simulink subsystem "ApplicationMotorSwapSysControl"  (R2024b)
settings: Solver=VariableStepAuto  StartTime=0.0  StopTime=10.0  RelTol=1e-3
values from neighbouring files (symbols this model uses):
  Ts = T_pwm    [mcbMotorSwapData.m]
  Ts_speed = 10*Ts    [mcbMotorSwapData.m]
undefined symbols (not defined in the file or in its folder): Per, Unit
libraries: simulink x2, mcbcomputeparameterlib x2, mcbcontrollergainlib x1
settings Model: Creator=The MathWorks, Inc.  LastModifiedBy=snarayan
settings RTWCC: GPUComputeCapability=3.5

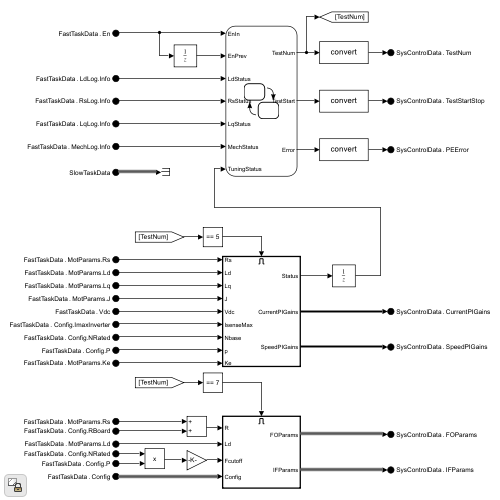
[thumbnail: Simulink's stored preview of the top-level diagram]
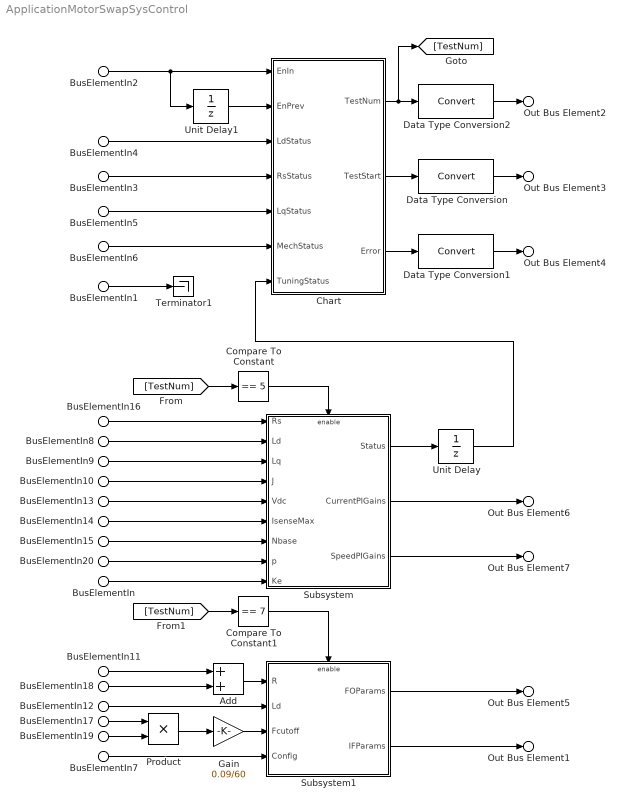
== system ApplicationMotorSwapSysControl ==
  BusElementIn2 : Inport  PortName=FastTaskData  Element=En
  BusElementIn3 : Inport  PortName=FastTaskData  Element=RsLog.Info
  BusElementIn4 : Inport  PortName=FastTaskData  Element=LdLog.Info
  BusElementIn5 : Inport  PortName=FastTaskData  Element=LqLog.Info
  BusElementIn6 : Inport  PortName=FastTaskData  Element=MechLog.Info
  BusElementIn11 : Inport  PortName=FastTaskData  Element=MotParams.Rs
  BusElementIn16 : Inport  PortName=FastTaskData  Element=MotParams.Rs
  BusElementIn8 : Inport  PortName=FastTaskData  Element=MotParams.Ld
  BusElementIn12 : Inport  PortName=FastTaskData  Element=MotParams.Ld
  BusElementIn9 : Inport  PortName=FastTaskData  Element=MotParams.Lq
  BusElementIn10 : Inport  PortName=FastTaskData  Element=MotParams.J
  BusElementIn : Inport  PortName=FastTaskData  Element=MotParams.Ke
  BusElementIn13 : Inport  PortName=FastTaskData  Element=Vdc
  BusElementIn7 : Inport  PortName=FastTaskData  Element=Config
  BusElementIn14 : Inport  PortName=FastTaskData  Element=Config.ImaxInverter
  BusElementIn15 : Inport  PortName=FastTaskData  Element=Config.NRated
  BusElementIn17 : Inport  PortName=FastTaskData  Element=Config.NRated
  BusElementIn18 : Inport  PortName=FastTaskData  Element=Config.RBoard
  BusElementIn19 : Inport  PortName=FastTaskData  Element=Config.P
  BusElementIn20 : Inport  PortName=FastTaskData  Element=Config.P
  BusElementIn1 : Inport  Port=2  PortName=SlowTaskData
  Add : Sum  RndMeth=Simplest  OutDataTypeStr=Inherit: Same as first input
  Chart : Stateflow chart  TreatAsAtomicUnit=on
  Compare To Constant : simulink/Logic and Bit Operations/Compare To Constant  relop===  const=5  OutDataTypeStr=boolean
  Compare To Constant1 : simulink/Logic and Bit Operations/Compare To Constant  relop===  const=7  OutDataTypeStr=boolean
  Data Type Conversion : DataTypeConversion  RndMeth=Simplest  SaturateOnIntegerOverflow=off
  Data Type Conversion1 : DataTypeConversion  RndMeth=Simplest  SaturateOnIntegerOverflow=off
  Data Type Conversion2 : DataTypeConversion  RndMeth=Simplest  SaturateOnIntegerOverflow=off
  Gain : Gain  Gain=0.09/60  RndMeth=Simplest  OutDataTypeStr=Inherit: Same as input
  Product : Product
  Subsystem : Subsystem
  Subsystem1 : Subsystem
  Terminator1 : Terminator
  Unit Delay : UnitDelay  SampleTime=-1  HasFrameUpgradeWarning=on
  Unit Delay1 : UnitDelay  SampleTime=-1  HasFrameUpgradeWarning=on
  Out Bus Element2 : Outport  PortName=SysControlData  Element=TestNum
  Out Bus Element3 : Outport  PortName=SysControlData  Element=TestStartStop
  Out Bus Element4 : Outport  PortName=SysControlData  Element=PEError
  Out Bus Element5 : Outport  PortName=SysControlData  Element=FOParams
  Out Bus Element6 : Outport  PortName=SysControlData  Element=CurrentPIGains
  Out Bus Element7 : Outport  PortName=SysControlData  Element=SpeedPIGains
  Out Bus Element1 : Outport  PortName=SysControlData  Element=IFParams
  wires:
  BusElementIn1/1 -> Terminator1/1
  BusElementIn2/1 -> Chart/1(EnIn), Unit Delay1/1
  Unit Delay1/1 -> Chart/2(EnPrev)
  Chart/1(TestNum) -> Data Type Conversion2/1, [TestNum]
  Chart/2(TestStart) -> Data Type Conversion/1
  BusElementIn3/1 -> Chart/4(RsStatus)
  BusElementIn4/1 -> Chart/3(LdStatus)
  BusElementIn5/1 -> Chart/5(LqStatus)
  BusElementIn6/1 -> Chart/6(MechStatus)
  Chart/3(Error) -> Data Type Conversion1/1
  BusElementIn8/1 -> Subsystem/2(Ld)
  BusElementIn9/1 -> Subsystem/3(Lq)
  BusElementIn10/1 -> Subsystem/4(J)
  Subsystem/1(Status) -> Unit Delay/1
  Unit Delay/1 -> Chart/7(TuningStatus)
  Data Type Conversion/1 -> Out Bus Element3/1
  Data Type Conversion1/1 -> Out Bus Element4/1
  Data Type Conversion2/1 -> Out Bus Element2/1
  BusElementIn11/1 -> Add/1
  BusElementIn12/1 -> Subsystem1/2(Ld)
  Subsystem1/1(FOParams) -> Out Bus Element5/1
  [TestNum] -> Compare To Constant/1
  Compare To Constant/1 -> Subsystem/Enable
  [TestNum] -> Compare To Constant1/1
  Compare To Constant1/1 -> Subsystem1/Enable
  Add/1 -> Subsystem1/1(R)
  BusElementIn13/1 -> Subsystem/5(Vdc)
  Product/1 -> Gain/1
  Gain/1 -> Subsystem1/3(Fcutoff)
  Subsystem/2(CurrentPIGains) -> Out Bus Element6/1
  Subsystem/3(SpeedPIGains) -> Out Bus Element7/1
  Subsystem1/2(IFParams) -> Out Bus Element1/1
  BusElementIn7/1 -> Subsystem1/4(Config)
  BusElementIn14/1 -> Subsystem/6(IsenseMax)
  BusElementIn15/1 -> Subsystem/7(Nbase)
  BusElementIn16/1 -> Subsystem/1(Rs)
  BusElementIn18/1 -> Add/2
  BusElementIn19/1 -> Product/2
  BusElementIn17/1 -> Product/1
  BusElementIn/1 -> Subsystem/9(Ke)
  BusElementIn20/1 -> Subsystem/8(p)

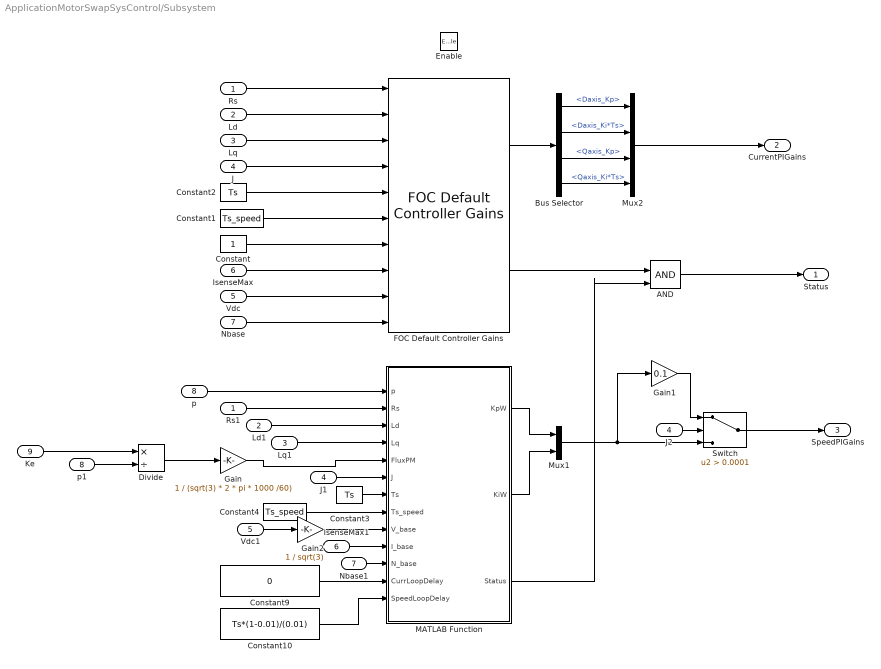
== system ApplicationMotorSwapSysControl/Subsystem ==
  Rs : Inport
  Ld : Inport  Port=2
  Lq : Inport  Port=3
  J : Inport  Port=4
  Vdc : Inport  Port=5
  IsenseMax : Inport  Port=6
  Nbase : Inport  Port=7
  p : Inport  Port=8
  Ke : Inport  Port=9
  Enable : EnablePort
  AND : Logic  IconShape=distinctive  AllPortsSameDT=off  OutDataTypeStr=boolean
  Bus Selector : BusSelector  OutputSignals=Daxis_Kp,Daxis_Ki*Ts,Qaxis_Kp,Qaxis_Ki*Ts
  Constant : Constant  OutDataTypeStr=dataType
  Constant1 : Constant  Value=Ts_speed  OutDataTypeStr=dataType
  Constant10 : Constant  Value=Ts*(1-0.01)/(0.01)  OutDataTypeStr=dataType
  Constant2 : Constant  Value=Ts  OutDataTypeStr=dataType
  Constant3 : Constant  Value=Ts  OutDataTypeStr=dataType
  Constant4 : Constant  Value=Ts_speed  OutDataTypeStr=dataType
  Constant9 : Constant  Value=0  OutDataTypeStr=dataType
  Divide : Product  Inputs=*/  RndMeth=Simplest  OutDataTypeStr=Inherit: Same as first input
  FOC Default Controller Gains : mcbcontrollergainlib/FOC Default Controller Gains  motorSelection=PMSM  unitType=Per-Unit  outCurrentControlGain=on  outFWCGain=off  outSpeedControlGain=on  externalDelay=off  currentSensorDelay=50e-6  speedSensorDelay=50e-6  speedFilterDelay=0.02
  Gain : Gain  Gain=1 / (sqrt(3) * 2 * pi * 1000 /60)  RndMeth=Simplest  OutDataTypeStr=Inherit: Same as input
  Gain1 : Gain  Gain=0.1  RndMeth=Simplest  OutDataTypeStr=Inherit: Same as input
  Gain2 : Gain  Gain=1 / sqrt(3)  RndMeth=Simplest  OutDataTypeStr=Inherit: Same as input
  IsenseMax1 : InportShadow  Port=6
  J1 : InportShadow  Port=4
  J2 : InportShadow  Port=4
  Ld1 : InportShadow  Port=2
  Lq1 : InportShadow  Port=3
  MATLAB Function : MATLAB Function  TreatAsAtomicUnit=on
  Mux1 : Mux  Inputs=2
  Mux2 : Mux
  Nbase1 : InportShadow  Port=7
  Rs1 : InportShadow
  Switch : Switch  Criteria=u2 > Threshold  Threshold=0.0001  SaturateOnIntegerOverflow=off  InputSameDT=off
  Vdc1 : InportShadow  Port=5
  p1 : InportShadow  Port=8
  Status : Outport
  CurrentPIGains : Outport  Port=2
  SpeedPIGains : Outport  Port=3
  wires:
  Gain1/1 -> Switch/1
  J2/1 -> Switch/2
  Switch/1 -> SpeedPIGains/1
  Bus Selector/4 -> Mux2/4  "<Qaxis_Ki*Ts>"
  Bus Selector/3 -> Mux2/3  "<Qaxis_Kp>"
  Bus Selector/2 -> Mux2/2  "<Daxis_Ki*Ts>"
  Bus Selector/1 -> Mux2/1  "<Daxis_Kp>"
  FOC Default Controller Gains/2 -> AND/1
  MATLAB Function/2(KiW) -> Mux1/2
  MATLAB Function/1(KpW) -> Mux1/1
  FOC Default Controller Gains/1 -> Bus Selector/1
  Gain2/1 -> MATLAB Function/9(V_base)
  AND/1 -> Status/1
  Vdc1/1 -> Gain2/1
  p1/1 -> Divide/2
  Ke/1 -> Divide/1
  p/1 -> MATLAB Function/1(p)
  Gain/1 -> MATLAB Function/5(FluxPM)
  Divide/1 -> Gain/1
  Nbase1/1 -> MATLAB Function/11(N_base)
  IsenseMax1/1 -> MATLAB Function/10(I_base)
  Constant4/1 -> MATLAB Function/8(Ts_speed)
  Constant3/1 -> MATLAB Function/7(Ts)
  J1/1 -> MATLAB Function/6(J)
  Lq1/1 -> MATLAB Function/4(Lq)
  Ld1/1 -> MATLAB Function/3(Ld)
  Rs1/1 -> MATLAB Function/2(Rs)
  Constant9/1 -> MATLAB Function/12(CurrLoopDelay)
  Constant10/1 -> MATLAB Function/13(SpeedLoopDelay)
  MATLAB Function/3(Status) -> AND/2
  Mux1/1 -> Gain1/1, Switch/3
  Mux2/1 -> CurrentPIGains/1
  Lq/1 -> FOC Default Controller Gains/3
  Nbase/1 -> FOC Default Controller Gains/10
  Vdc/1 -> FOC Default Controller Gains/9
  J/1 -> FOC Default Controller Gains/4
  Ld/1 -> FOC Default Controller Gains/2
  Constant2/1 -> FOC Default Controller Gains/5
  Constant/1 -> FOC Default Controller Gains/7
  IsenseMax/1 -> FOC Default Controller Gains/8
  Constant1/1 -> FOC Default Controller Gains/6
  Rs/1 -> FOC Default Controller Gains/1

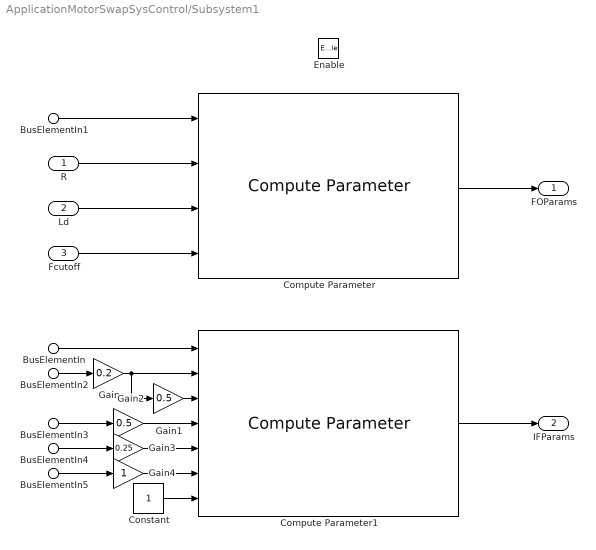
== system ApplicationMotorSwapSysControl/Subsystem1 ==
  R : Inport
  Ld : Inport  Port=2
  Fcutoff : Inport  Port=3
  BusElementIn : Inport  Port=4  PortName=Config  Element=P
  BusElementIn1 : Inport  Port=4  PortName=Config  Element=P
  BusElementIn2 : Inport  Port=4  PortName=Config  Element=NRated
  BusElementIn4 : Inport  Port=4  PortName=Config  Element=NRated
  BusElementIn3 : Inport  Port=4  PortName=Config  Element=IRated
  BusElementIn5 : Inport  Port=4  PortName=Config  Element=IRated
  Enable : EnablePort
  Compute Parameter : mcbcomputeparameterlib/Compute Parameter  PathOfCompatibleBlock=Microcontroller/ApplicationFastTask/FluxObserver/Flux Observer
  Compute Parameter1 : mcbcomputeparameterlib/Compute Parameter  PathOfCompatibleBlock=Microcontroller/ApplicationFastTask/FOCRun/IFController/I-F Controller
  Constant : Constant  OutDataTypeStr=dataType
  Gain : Gain  Gain=0.2  RndMeth=Simplest  OutDataTypeStr=Inherit: Same as input
  Gain1 : Gain  Gain=0.5  RndMeth=Simplest  OutDataTypeStr=Inherit: Same as input
  Gain2 : Gain  Gain=0.5  RndMeth=Simplest  OutDataTypeStr=Inherit: Same as input
  Gain3 : Gain  Gain=0.25  RndMeth=Simplest  OutDataTypeStr=Inherit: Same as input
  Gain4 : Gain  RndMeth=Simplest  OutDataTypeStr=Inherit: Same as input
  FOParams : Outport
  IFParams : Outport  Port=2
  wires:
  Gain4/1 -> Compute Parameter1/6
  BusElementIn5/1 -> Gain4/1
  Constant/1 -> Compute Parameter1/7
  BusElementIn4/1 -> Gain3/1
  Gain3/1 -> Compute Parameter1/5
  Gain2/1 -> Compute Parameter1/4
  BusElementIn3/1 -> Gain2/1
  Gain1/1 -> Compute Parameter1/3
  Gain/1 -> Gain1/1, Compute Parameter1/2
  BusElementIn2/1 -> Gain/1
  Compute Parameter1/1 -> IFParams/1
  BusElementIn/1 -> Compute Parameter1/1
  BusElementIn1/1 -> Compute Parameter/1
  Ld/1 -> Compute Parameter/3
  Compute Parameter/1 -> FOParams/1
  Fcutoff/1 -> Compute Parameter/4
  R/1 -> Compute Parameter/2

== matlab function ApplicationMotorSwapSysControl/Subsystem/MATLAB Function ==
  data: p input; KpW output; KiW output; Rs input; Ld input; Lq input; FluxPM input; J input; Ts input; Ts_speed input; V_base input; I_base input; N_base input; CurrLoopDelay input; SpeedLoopDelay input; Status output
function [KpW, KiW, Status] = fcn(p,Rs,Ld,Lq,FluxPM,J,Ts,Ts_speed,V_base,I_base,N_base,CurrLoopDelay,SpeedLoopDelay)

if (p<=0 || Rs<=0 || Ld<=0 || Lq<=0 || FluxPM<=0 || J<=0 || Ts<=0 || Ts_speed<=0 || V_base<=0 || I_base<=0 || N_base<=0 || CurrLoopDelay<0 || SpeedLoopDelay<0)
    Status = false;    
    
    KpW = single (0);
    KiW = single (0);
else
    Status = true; % Output is ok
    %% D-axis current loop
    % Define plant
    DCLPlant.Gain = V_base/(I_base*Rs);
    DCLPlant.TimeConstant = Ld/Rs;
    % Define delay components in forward path
    DCLForwardPathDelay.Gain = cast(1,'like',Ts);
    DCLForwardPathDelay.TimeConstant = Ts/2;
    % Define delay components in feedback path
    DCLFeedbackPathDelay.Gain = [cast(1,'like',Ts) cast(1,'like',Ts)];
    DCLFeedbackPathDelay.TimeConstant = [Ts/2 CurrLoopDelay];
    % calculate gain using modulus optimum theory
    [DCLPIGains,~,~] = calcControllerGain(DCLPlant,DCLForwardPathDelay,DCLFeedbackPathDelay,'Modulus',cast(1,'like',Ts));

    %% Q-axis current loop
    % Define plant
    QCLPlant.Gain = V_base/(I_base*Rs);
    QCLPlant.TimeConstant = Lq/Rs;
    % Define delay components in forward path
    QCLForwardPathDelay.Gain = cast(1,'like',Ts);
    QCLForwardPathDelay.TimeConstant = Ts/2;
    % Define delay components in feedback path
    QCLFeedbackPathDelay.Gain = [cast(1,'like',Ts) cast(1,'like',Ts)];
    QCLFeedbackPathDelay.TimeConstant = [Ts/2 CurrLoopDelay];
    % calculate gain using modulus optimum theory
    [QCLPIGains,~,QCLDelay] = calcControllerGain(QCLPlant,QCLForwardPathDelay,QCLFeedbackPathDelay,'Modulus',cast(1,'like',Ts));

    %% Speed loop
    % Define plant
    SLPlant.Gain = (cast(60,'like',Ts)*cast(1.5,'like',Ts)*p*FluxPM*I_base)/(2*cast(pi,'like',Ts)*N_base*J);
    SLPlant.TimeConstant = 0;
    % Define delay components in forward path
    SLForwardPathDelay.Gain = [cast(1,'like',Ts) QCLDelay(1)];
    SLForwardPathDelay.TimeConstant = [Ts_speed/2 QCLDelay(2)];
    % Define delay components in feedback path
    SLFeedbackPathDelay.Gain = [cast(1,'like',Ts) cast(1,'like',Ts)];
    SLFeedbackPathDelay.TimeConstant = [Ts_speed/2 SpeedLoopDelay];
    % calculate gain using symmetric optimum theory and multiply with scaling factor
    [SLPIGains,~,~] = calcControllerGain(SLPlant,SLForwardPathDelay,SLFeedbackPathDelay,'Symmetric',cast(1,'like',Ts));
    
    
    KpW = SLPIGains.Kp;
    KiW = SLPIGains.Ki * Ts_speed;
end

== stateflow chart ApplicationMotorSwapSysControl/Chart ==
  state Init
    during:
    TestNum = uint16(0);
    TestStart = false;
    Error = single(0);
  state Rs
    during:
    TestNum = uint16(1);
    TestStart = true;
  state Error
    during:
    TestNum = uint16(0);
    TestStart = false;
  state Ld
    during:
    TestNum = uint16(2);
    TestStart = true;
  state Lq
    during:
    TestNum = uint16(3);
    TestStart = true;
  state FOTune
    during:
    TestNum = uint16(7);
    TestStart = false;
    Error = single(0);
  state Mech
    during:
    TestNum = uint16(4);
    TestStart = true;
  state PITuning
    during:
    TestNum = uint16(5);
    TestStart = false;
  state ClosedLoopRun
    during:
    TestNum = uint16(6);
    TestStart = true;
  (default) -> Init
  Rs -> Error [order 2] : [RsStatus > 2]{Error = RsStatus;}
  Init -> Rs : [EnIn == true && EnPrev == false]
  Rs -> Ld [order 1] : after(0.5,sec)[RsStatus == 2]
  Ld -> Error [order 2] : [LdStatus > 2]{Error = LdStatus;}
  Ld -> Lq [order 1] : after(0.5,sec)[LdStatus == 2]
  Lq -> FOTune [order 2] : after(0.5,sec)[LqStatus == 2]
  Lq -> Error [order 1] : [LqStatus > 2]{Error = LqStatus;}
  FOTune -> Mech : after(0.5,sec)
  Mech -> Error [order 1] : [MechStatus > 2]{Error = MechStatus;}
  Mech -> PITuning [order 2] : after(0.5,sec)[MechStatus == 2]
  PITuning -> ClosedLoopRun : after(0.5,sec)[TuningStatus == 1]
  data: EnIn input; EnPrev input; TestNum output uint16; TestStart output boolean; LdStatus input; RsStatus input; LqStatus input; MechStatus input; Error output single; TuningStatus input
